simulink model "third"  (R2018a)
settings: Solver=VariableStepAuto  StartTime=0.0  StopTime=10.0  RelTol=1e-3
values from neighbouring files (symbols this model uses):
  kd = 0.2    [matlab.mat]
  Qs = 0.125    [matlab.mat]
  R = 1.6    [matlab.mat]
settings Model: Creator=Master  LastModifiedBy=Master

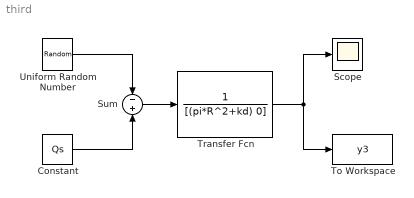
== system third ==
  Constant : Constant  Value=Qs
  Scope : Scope
  Sum : Sum  Inputs=-|+
  To Workspace : ToWorkspace  VariableName=y3  SaveFormat=Timeseries  SampleTime=-1
  Transfer Fcn : TransferFcn  Denominator=[(pi*R^2+kd) 0]
  Uniform Random Number : UniformRandomNumber  SampleTime=0.1
  wires:
  Uniform Random Number/1 -> Sum/1
  Constant/1 -> Sum/2
  Sum/1 -> Transfer Fcn/1
  Transfer Fcn/1 -> To Workspace/1, Scope/1
